simulink model "Dynamics_PID_ADAMS"  (R2022a)
settings: Solver=FixedStepAuto  StartTime=0.0  StopTime=5  FixedStep=0.001  RelTol=1e-3
undefined symbols (not defined in the file): ADAMS_cwd, ADAMS_exec, ADAMS_host, ADAMS_init, ADAMS_inputs, ADAMS_outputs, ADAMS_prefix, ADAMS_static, ADAMS_sysdir
settings Model: Creator=moham  LastModifiedBy=Mohammed Ashraf

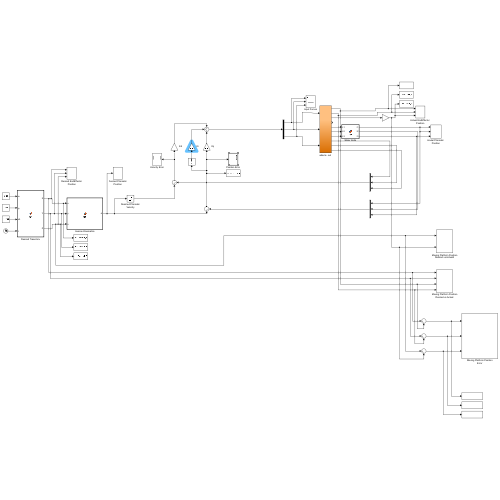
[thumbnail: Simulink's stored preview of the top-level diagram]
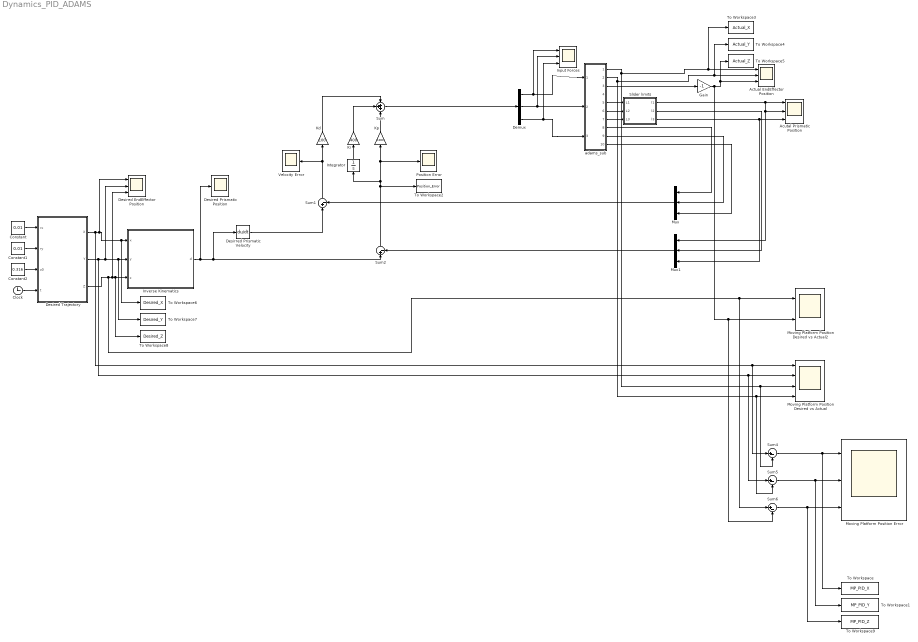
== system Dynamics_PID_ADAMS ==
  Actual EndEffector Position : Scope  NumInputPorts=3
  Acutal Prismatic Position : Scope  NumInputPorts=3
  Clock : Clock
  Constant : Constant  Value=0.01
  Constant1 : Constant  Value=0.01
  Constant2 : Constant  Value=0.316
  Demux : Demux  Outputs=3
  Desired EndEffector Position : Scope  NumInputPorts=3
  Desired Prismatic Position : Scope
  Desired Trajectory : MATLAB Function  TreatAsAtomicUnit=on
  Desirred Prismatic Velocity : Derivative
  Gain : Gain  Gain=-1
  Input Forces : Scope  NumInputPorts=3
  Integrator : Integrator
  Inverse Kinematics : MATLAB Function  TreatAsAtomicUnit=on
  Kd : Gain  Gain=100
  Ki : Gain  Gain=400
  Kp : Gain  Gain=1000
  Moving Platform Position Desired vs Actual : Scope  NumInputPorts=4
  Moving Platform Position Desired vs Actual2 : Scope  NumInputPorts=2
  Moving Platform Position Error : Scope  NumInputPorts=3
  Mux : Mux  Inputs=3
  Mux1 : Mux  Inputs=3
  Position Error : Scope
  Slider limits : MATLAB Function  TreatAsAtomicUnit=on
  Sum : Sum  Inputs=3
  Sum{1..2,4..6} (5 alike) : Sum  Inputs=|+-
  To Workspace : ToWorkspace  VariableName=MP_PID_X  SampleTime=-1
  To Workspace1 : ToWorkspace  VariableName=MP_PID_Y  SampleTime=-1
  To Workspace2 : ToWorkspace  VariableName=Position_Error  SampleTime=-1
  To Workspace3 : ToWorkspace  VariableName=Actual_X  SampleTime=-1
  To Workspace4 : ToWorkspace  VariableName=Actual_Y  SampleTime=-1
  To Workspace5 : ToWorkspace  VariableName=Actual_Z  SampleTime=-1
  To Workspace6 : ToWorkspace  VariableName=Desired_X  SampleTime=-1
  To Workspace7 : ToWorkspace  VariableName=Desired_Y  SampleTime=-1
  To Workspace8 : ToWorkspace  VariableName=Desired_Z  SampleTime=-1
  To Workspace9 : ToWorkspace  VariableName=MP_PID_Z  SampleTime=-1
  Velocity Error : Scope
  adams_sub : Subsystem
  wires:
  adams_sub/7("Position3            ") -> Slider limits/3(L3)
  adams_sub/10("Velocity3            ") -> Mux/3
  adams_sub/9("Velocity2            ") -> Mux/2
  Desirred Prismatic Velocity/1 -> Sum1/1
  Sum1/1 -> Velocity Error/1, Kd/1
  Demux/3 -> adams_sub/3(Force3), Input Forces/3
  Mux1/1 -> Sum2/2
  Slider limits/3(l3) -> Mux1/3, Acutal Prismatic Position/3
  Clock/1 -> Desired Trajectory/4(t)
  Mux/1 -> Sum1/2
  Slider limits/1(l1) -> Acutal Prismatic Position/1, Mux1/1, Acutal Prismatic Position/2
  Slider limits/2(l2) -> Mux1/2
  adams_sub/6("Position2            ") -> Slider limits/2(L2)
  adams_sub/5("Position1            ") -> Slider limits/1(L1)
  Demux/2 -> adams_sub/2(Force2), Input Forces/2
  Constant2/1 -> Desired Trajectory/3(z0)
  Constant1/1 -> Desired Trajectory/2(ry)
  Sum2/1 -> To Workspace2/1, Integrator/1, Kp/1, Position Error/1
  Constant/1 -> Desired Trajectory/1(rx)
  Demux/1 -> adams_sub/1(Force1), Input Forces/1
  adams_sub/8("Velocity1            ") -> Mux/1
  Inverse Kinematics/1(d) -> Desired Prismatic Position/1, Desirred Prismatic Velocity/1, Sum2/1
  Kd/1 -> Sum/1
  Sum/1 -> Demux/1
  Kp/1 -> Sum/3
  Integrator/1 -> Ki/1
  Ki/1 -> Sum/2
  Desired Trajectory/3(Z) -> Sum6/1, Moving Platform Position Desired vs Actual2/1, Desired EndEffector Position/3, To Workspace8/1, Inverse Kinematics/3(z)
  Desired Trajectory/2(Y) -> Sum5/1, Moving Platform Position Desired vs Actual/2, Desired EndEffector Position/2, To Workspace7/1, Inverse Kinematics/2(y)
  adams_sub/2(EndEffector_YPosition) -> Sum5/2, Moving Platform Position Desired vs Actual/4, To Workspace4/1, Actual EndEffector Position/2
  Sum4/1 -> To Workspace/1, Moving Platform Position Error/1
  Sum6/1 -> To Workspace9/1, Moving Platform Position Error/3
  Desired Trajectory/1(X) -> Sum4/1, Moving Platform Position Desired vs Actual/1, Desired EndEffector Position/1, To Workspace6/1, Inverse Kinematics/1(x)
  Sum5/1 -> To Workspace1/1, Moving Platform Position Error/2
  adams_sub/1(EndEffector_XPosition) -> Sum4/2, Moving Platform Position Desired vs Actual/3, To Workspace3/1, Actual EndEffector Position/1
  Gain/1 -> Sum6/2, Moving Platform Position Desired vs Actual2/2, To Workspace5/1, Actual EndEffector Position/3
  adams_sub/3(EndEffector_ZPosition) -> Gain/1

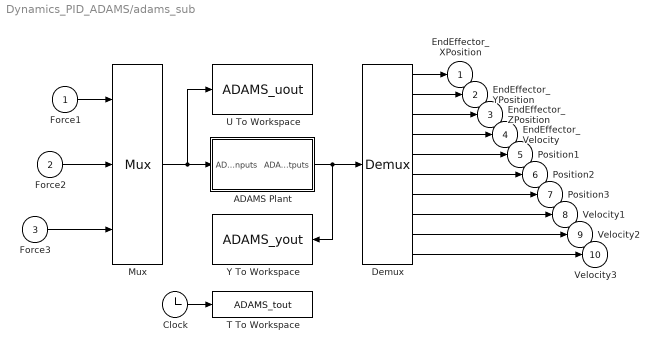
== system Dynamics_PID_ADAMS/adams_sub ==
  Force1 : Inport
  Force2 : Inport  Port=2
  Force3 : Inport  Port=3
  ADAMS Plant : Subsystem  LoadFcn=|  InitFcn=clear mex  mask(Adams Plant){exevie=ADAMS_sysdir, nam_in=ADAMS_inputs, namout=ADAMS_outputs, nampre=ADAMS_prefix, outfil=ADAMS_prefix, exesol=ADAMS_exec, stat=ADAMS_static, inicmd=[ADAMS_init], exetyp=C++, comtyp=PIPE(DDE), workdir=ADAMS_cwd, ada_host=ADAMS_host, modani=batch, modsim=discrete, dft=no, simulink_lead_cosim=yes, pin_interp_order=0, pout_extrap_order=0, pin_extrap_order=0, pout_interp_order=0, dt_out=0.005, o_rate=1, more=off}
      | %check based on dialog box setting for when setting by popup menu                                             
      | if exist('ADAMS_solver_type')                                                                                 
      |   if strcmp(ADAMS_solver_type,'C++')                                                                          
      |     set_param(gcb,'exetyp','C++');                                                                            
      |   else                                                                                                        
      |     set_param(gcb,'exetyp','Fortran');                                                                        
      |   end                                                                                                         
      | else                                                                                                          
      |   set_param(gcb,'exetyp','C++');                                                                              
      | end                                                                                                           
      | %set the mode if using acar_solver                                                                            
      | %REQUIRED HERE BECAUSE BELOW CAUSES MDLTERMINATE TO BE CALLED 2 TIMES IN MIDDLE OF SIMULATION WHEN SET IN MASK
      |                                                                                                               
      | %enable the direct feedthrough, sim mode, anim mode parameters by default                                     
      |                                                                                                               
      | if exist('set_some_params_states')                                                                            
      |                                                                                                               
      |   set_some_params_states({'dft','modsim','modani'},{'on','on','on'},'MaskEnables',gcb)                        
      |   %turn on direct feedthrough option                                                                          
      |   set_some_params_states({'dft'},{'on'},'MaskVisibilities',gcb)                                               
      |                                                                                                               
      |  end                                                                                                          
      |                                                                                                               
      |                                                                                                               
      | if exist('ADAMS_exec')                                                                                        
      |   if and(strcmp(get_param(gcb,'exesol'),'ADAMS_exec'),strcmp(ADAMS_exec,'acar_solver'))                       
      |     %set the sim mode to discrete -- only supported mode                                                      
      |     set_param(gcb,'modsim','discrete')                                                                        
      |      %turn off direct feedthrough option                                                                      
      |      set_some_params_states({'dft'},{'off'},'MaskVisibilities',gcb)                                           
      |     %set the animation mode to batch -- only supported mode                                                   
      |     set_param(gcb,'modani','batch')                                                                           
      |     %disable the direct feedthrough, sim mode, anim mode parameters                                           
      |     set_some_params_states({'modsim','modani'},{'off','off'},'MaskEnables',gcb)                               
      |   end
      |   if and(strcmp(get_param(gcb,'exesol'),'ADAMS_exec'),strcmp(ADAMS_exec,'apre_solver'))                       
      |     %set the sim mode to discrete -- only supported mode                                                      
      |     set_param(gcb,'modsim','discrete')                                                                        
      |      %turn off direct feedthrough option                                                                      
      |      set_some_params_states({'dft'},{'off'},'MaskVisibilities',gcb)                                           
      |     %set the animation mode to batch -- only supported mode                                                   
      |     set_param(gcb,'modani','batch')                                                                           
      |     %disable the direct feedthrough, sim mode, anim mode parameters                                           
      |     set_some_params_states({'modsim','modani'},{'off','off'},'MaskEnables',gcb)                               
      |   end                                                                                                  
      | end
      mask prompts: exevie "Adams install directory"; nam_in "Adams View input names"; namout "Adams View output names"; nampre "Adams model file prefix"; outfil "Output files prefix (opt.: if blank - no output)"; exesol "User executable (opt.: if blank - use standard)"; stat "Initial static simulation flag"; inicmd "Initialization commands"; exetyp "Adams Solver type"; comtyp "Interprocess option"; workdir "Adams working directory"; ada_host "Adams host"; modani "Animation mode"; modsim "Simulation mode"; dft "Direct feedthrough"; simulink_lead_cosim "Discrete Computational Order - Simulink Leads Adams"; pin_interp_order "Plant input interpolation order"; pout_extrap_order "Plant output extrapolation order"; pin_extrap_order "Plant input extrapolation order"; pout_interp_order "Plant output interpolation order"; dt_out "Communication interval"; o_rate "Number of communications per output step"; more "More parameters"
      mask help: Simulate any Adams plant model either in Adams Solver form (.adm file) or in Adams View form (.cmd file)
      settings: OpenFcn=|
      | open_system(gcb,'mask')
      | if not(exist('set_some_params_states'))
      | 
      | warning('The script "set_some_params_states.m" cannot be found in the MATLAB PATH.  Cannot update the ADAMS Plant S-Function parameters.')
      | 
      | warning('Recommended action(optional):  run the Adams Controls .m file first to help choose the correct settings in the Adams S-Function block.')
      | 
      | end
      mask Help:
      | <html>
      | This S-Function represents the non-linear Adams Plant with the inputs sent to the Adams model <br>
      |  and the outputs generated by the Adams model.  See the Adams Controls documentation for more <br>
      | information.  This plant uses the following variables:<br>
      | <br>
      | <b>ADAMS_sysdir  :</b> Adams installation directory<br>
      | <b>ADAMS_inputs  :</b> Input variables View names vector<br>
      | <b>ADAMS_outputs :</b> Outputs variables View names vector<br>
      | <b>ADAMS_prefix  : </b>ADAMS model files prefix (.adm, .cmd); also doubles as output files prefix<br>
      | <b>ADAMS_exec :</b> Adams Solver user library or keyword (e.g., acar_solver)<br>
      | <b>ADAMS_static :</b> yes|no - initial static before Co-simulation(discrete)/Function Evaluation(continuous)<br>
      | <b>ADAMS_init :</b>Initialization commands (i.e., Adams View or Solver commands, depending on setting for Animation mode)<br>
      | <b>ADAMS_cwd : </b> Current working directory (for TCP/IP)<br>
      | <b>ADAMS_host : </b>Name of Adams server host (for TCP/IP)<br>
      | <b>ADAMS_mode :</b> Linear or non-linear (i.e., co-sim, function eval)<br>
      | <b>ADAMS_solver_type :</b>Fortran or C++ (used to set popup menu when first loaded) <br>
      | 
      | 
      | <br>
      | The following settings can be chosen:<br>
      | <br>
      | <b>Adams Solver type:</b>  Fortran or C++ (will also set ADAMS_solver_type)<br>
      | <b>Interprocess option:</b> Pipe(DDE), TCP/IP or DIRECT; TCP/IP can allow different machines run Adams and MATLAB<br>
      | <b>Animation mode:</b> batch (Solver, uses .adm) or interactive (View, uses .cmd)<br>
      | <b>Simulation mode:</b> discrete (Co-simulation) or continuous (Function Evaluation)<br>
      | <b>Discrete Computational Order - Simulink Lead Adams:</b> for discrete mode, chooses if Simulink leads the integration (yes) or lags (no);<br> if set to "no", can remove algebraic loop<br>
      | <b>Plant input interpolation order:</b> 0 = zero-order hold; 1 = linear (discrete mode only, where Simulink leads)<br>
      | <b>Plant output extrapolation order:</b> 0 = zero-order hold;1 = linear(discrete mode only, where Simulink leads)<br>
      | <b>Plant input extrapolation order:</b> 0 = zero-order hold; 1 = linear (discrete mode only, where Adams leads)<br>
      | <b>Plant output interpolation order:</b> 0 = zero-order hold;1 = linear(discrete mode only, where Adams leads)<br>
      | <b>Direct feedthrough:</b> yes|no - yes = Input directly effect output(continuous mode-only)<br>
      | <b>Communication interval:</b> Time step at which Co-simulation exchange information (e.g.,0.005); also controls <br>output for continuous mode (Function Evaluation)<br>
      | <b>Number of communications per output step: </b>Sets Adams output rate (.res, .req, .gra) integer value (default: 1)<br>
      | </html>
      mask Callback exesol:
      | if exist('set_some_params_states')
      | %enable the direct feedthrough, sim mode, anim mode parameters
      | set_some_params_states({'dft','modsim','modani'},{'on','on','on'},'MaskEnables',gcb)
      | %turn on direct feedthrough option
      | set_some_params_states({'dft'},{'on'},'MaskVisibilities',gcb)
      | end
      | 
      | if exist('ADAMS_exec')
      |   if and(strcmp(get_param(gcb,'exesol'),'ADAMS_exec'),strcmp(ADAMS_exec,'acar_solver'))
      |     %set the sim mode to discrete -- only supported mode
      |     %REMOVED:  BELOW CAUSES MDLTERMINATE TO BE CALLED 2 TIMES IN MIDDLE OF SIMULATION
      |     %Now in LoadFcn callback
      |     %set_param(gcb,'modsim','discrete')
      |      %turn off direct feedthrough option
      |     set_some_params_states({'dft'},{'off'},'MaskVisibilities',gcb)
      |     %set the animation mode to batch -- only supported mode
      |     %REMOVED:  BELOW CAUSES MDLTERMINATE TO BE CALLED 2 TIMES IN MIDDLE OF SIMULATION
      |     %Now in LoadFcn callback
      |     %set_param(gcb,'modani','batch')
      |     %disable the direct feedthrough, sim mode, anim mode parameters
      |     set_some_params_states({'modsim','modani'},{'off','off'},'MaskEnables',gcb)
      |   end
      | end
      mask TypeOptions exetyp: Fortran | C++
      mask Callback exetyp:
      | if strcmp(get_param(gcb,'exetyp'),'C++')
      |     ADAMS_solver_type='C++';
      | else
      |     ADAMS_solver_type='Fortran';
      | end
      mask TypeOptions comtyp: PIPE(DDE) | TCP/IP | DIRECT
      mask Callback comtyp:
      | if exist('set_some_params_states')
      | if strcmp(get_param(gcb,'comtyp'),'PIPE(DDE)') || strcmp(get_param(gcb,'comtyp'),'DIRECT')
      |     %turn off cwd, host options
      |     set_some_params_states({'ada_host','workdir'},{'off','off'},'MaskVisibilities',gcb)
      | else%if strcmp(get_param(gcb,'modsim'),'TCP/IP')
      |     %turn on cwd, host options
      |     set_some_params_states({'ada_host','workdir'},{'on','on'},'MaskVisibilities',gcb)
      | end
      | end
      mask TypeOptions modani: batch | interactive
      mask TypeOptions modsim: discrete | continuous
      mask Callback modsim:
      | if exist('set_some_params_states')
      | if strcmp(get_param(gcb,'modsim'),'discrete')
      |      %turn off direct feedthrough option
      |     set_some_params_states({'dft'},{'off'},'MaskVisibilities',gcb)
      |     %turn on discrete co-sim type if want to see more
      |     if strcmp(get_param(gcb,'more'),'on')
      |         set_some_params_states({'simulink_lead_cosim'},{'on'},'MaskVisibilities',gcb)
      |     end
      |     if strcmp(get_param(gcb,'simulink_lead_cosim'),'yes')
      |         %turn on interpolation/extrapolation options
      |         set_some_params_states({'pin_interp_order','pout_extrap_order',},{'on','on'},'MaskVisibilities',gcb)
      |     else
      |         set_some_params_states({'pin_extrap_order','pout_interp_order'},{'on','on'},'MaskVisibilities',gcb)
      |     end
      | else%if strcmp(get_param(gcb,'modsim'),'continuous')
      |      %turn off direct feedthrough option
      |     set_some_params_states({'dft'},{'on'},'MaskVisibilities',gcb)
      |     %turn off interpolation/extrapolation options
      |     set_some_params_states({'pin_interp_order','pout_extrap_order','pin_extrap_order','pout_interp_order','simulink_lead_cosim'},{'off','off','off','off','off'},'MaskVisibilities',gcb)
      | end
      | end
      mask TypeOptions dft: no | yes
      mask TypeOptions simulink_lead_cosim: yes | no
      mask Callback simulink_lead_cosim:
      | if exist('set_some_params_states')
      | if (strcmp(get_param(gcb,'simulink_lead_cosim'),'yes') && strcmp(get_param(gcb,'modsim'),'discrete'))
      |      %turn off unused interpolate/extrapolate options
      |     set_some_params_states({'pin_extrap_order','pout_interp_order'},{'off','off'},'MaskVisibilities',gcb)
      |     %turn on used interpolate/extrapolate options
      |     set_some_params_states({'pin_interp_order','pout_extrap_order'},{'on','on'},'MaskVisibilities',gcb)
      | elseif (strcmp(get_param(gcb,'simulink_lead_cosim'),'no') && strcmp(get_param(gcb,'modsim'),'discrete'))
      |     %turn on used interpolate/extrapolate options
      |     set_some_params_states({'pin_extrap_order','pout_interp_order'},{'on','on'},'MaskVisibilities',gcb)
      |      %turn off unused interpolate/extrapolate options
      |     set_some_params_states({'pin_interp_order','pout_extrap_order'},{'off','off'},'MaskVisibilities',gcb)
      | end
      | end
      mask TypeOptions pin_interp_order: 0 | 1
      mask TypeOptions pout_extrap_order: 0 | 1
      mask TypeOptions pin_extrap_order: 0 | 1
      mask TypeOptions pout_interp_order: 0 | 1
      mask Callback more:
      | if exist('set_some_params_states')
      | if (strcmp(get_param(gcb,'more'),'on'))
      |      %turn on infrequently used options
      |     set_some_params_states({'exevie','nam_in','namout','exesol','stat','inicmd'},{'on','on','on','on','on','on'},'MaskVisibilities',gcb)
      |     if strcmp(get_param(gcb,'modsim'),'discrete')
      |         set_some_params_states({'simulink_lead_cosim'},{'on'},'MaskVisibilities',gcb)
      |     end
      | elseif (strcmp(get_param(gcb,'more'),'off'))
      |     %turn off infrequently used options
      |     set_some_params_states({'exevie','nam_in','namout','exesol','stat','inicmd'},{'off','off','off','off','off','off'},'MaskVisibilities',gcb)
      |     if strcmp(get_param(gcb,'modsim'),'discrete')
      |         set_some_params_states({'simulink_lead_cosim'},{'off'},'MaskVisibilities',gcb)
      |     end
      | end
      | end
      mask Display: disp( 'MSC Software' )
  Clock : Clock
  Demux : Demux  Outputs=10
      settings: DisplayOption=none
  Mux : Mux  Inputs=3
  T To Workspace : ToWorkspace  VariableName=ADAMS_tout
      settings: MaxDataPoints=100000
  U To Workspace : ToWorkspace  VariableName=ADAMS_uout
      settings: MaxDataPoints=100000
  Y To Workspace : ToWorkspace  VariableName=ADAMS_yout
      settings: MaxDataPoints=100000
  EndEffector_XPosition : Outport
  EndEffector_YPosition : Outport  Port=2
  EndEffector_ZPosition : Outport  Port=3
  "EndEffector_Velocity " : Outport  Port=4
  "Position1            " : Outport  Port=5
  "Position2            " : Outport  Port=6
  "Position3            " : Outport  Port=7
  "Velocity1            " : Outport  Port=8
  "Velocity2            " : Outport  Port=9
  "Velocity3            " : Outport  Port=10
  wires:
  Clock/1 -> T To Workspace/1
  Mux/1 -> ADAMS Plant/1(ADAMS inputs), U To Workspace/1
  ADAMS Plant/1(ADAMS outputs) -> Demux/1, Y To Workspace/1
  Demux/1 -> EndEffector_XPosition/1
  Demux/2 -> EndEffector_YPosition/1
  Demux/3 -> EndEffector_ZPosition/1
  Demux/4 -> "EndEffector_Velocity "/1
  Demux/5 -> "Position1            "/1
  Demux/6 -> "Position2            "/1
  Demux/7 -> "Position3            "/1
  Demux/8 -> "Velocity1            "/1
  Demux/9 -> "Velocity2            "/1
  Demux/10 -> "Velocity3            "/1
  Force1/1 -> Mux/1
  Force2/1 -> Mux/2
  Force3/1 -> Mux/3

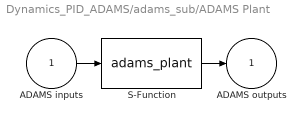
== system Dynamics_PID_ADAMS/adams_sub/ADAMS Plant ==
  ADAMS inputs : Inport
  S-Function : S-Function  StopFcn=clear mex  FunctionName=adams_plant  Parameters=exevie,exesol,stat,outfil,nampre,o_rate,nam_in,namout,dft,modsim,modani,dt_out,inicmd,exetyp,comtyp,ada_host, workdir,pin_interp_order,pout_extrap_order,pin_extrap_order,pout_interp_order,simulink_lead_cosim  SFunctionDeploymentMode=off  EnableBusSupport=off
  ADAMS outputs : Outport  InitialOutput=0
  wires:
  ADAMS inputs/1 -> S-Function/1
  S-Function/1 -> ADAMS outputs/1

== matlab function Dynamics_PID_ADAMS/Inverse Kinematics ==
  data: x input; d output; y input; z input
function d = fcn(x,y,z)
SB = 0.485; % meters
WB = 0.140; % meters
UB = 0.280; % meters

sp = 0.09268;
wp = 0.02675;
up = 0.05351;

l = 0.365; % meters

a = SB/2 - sp/2;
b = WB - wp;
c = up - UB;

C1 = x^2 + y^2 + z^2 + a^2 + b^2 + 2*a*x + 2*b*y - l^2;
C2 = x^2 + y^2 + z^2 + a^2 + b^2 - 2*a*x + 2*b*y - l^2 ;
C3 = x^2 + y^2 + z^2 + c^2 + 2*c*y - l^2;

L1 = -z - (z^2 - C1)^0.5 - 0.054; % adding 5 cm offset for prismatic joint width
L2 = -z - (z^2 - C2)^0.5 - 0.054; % adding 5 cm offset for prismatic joint width
L3 = -z - (z^2 - C3)^0.5 - 0.054; % adding 5 cm offset for prismatic joint width

d = [L1; L2; L3];

end

== matlab function Dynamics_PID_ADAMS/Desired Trajectory ==
  data: X output; rx input; Y output; ry input; z0 input; t input; Z output
function [X,Y,Z] = fcn(rx, ry, z0, t)

w = 1;
v = 1;


X =  rx*sin((pi/6)*t);
Y =  ry*cos((pi/6)*t);
Z = -(z0 + ((pi/6)*t)/100);

end

== matlab function Dynamics_PID_ADAMS/Slider limits ==
  data: L1 input; l1 output; L2 input; L3 input; l2 output; l3 output
function [l1, l2, l3] = fcn(L1, L2, L3)


l1 = L1;
l2 = L2;
l3 = L3;

end
